simulink model "time_test"  (R2018b)
settings: Solver=VariableStepAuto  StartTime=0.0  StopTime=0  FixedStep=.2  RelTol=1e-3
values from neighbouring files (symbols this model uses):
  utc_test = 137803367    [time_test_init.m]
libraries: time_lib x1
settings Model: Creator=devantormey  LastModifiedBy=devantormey

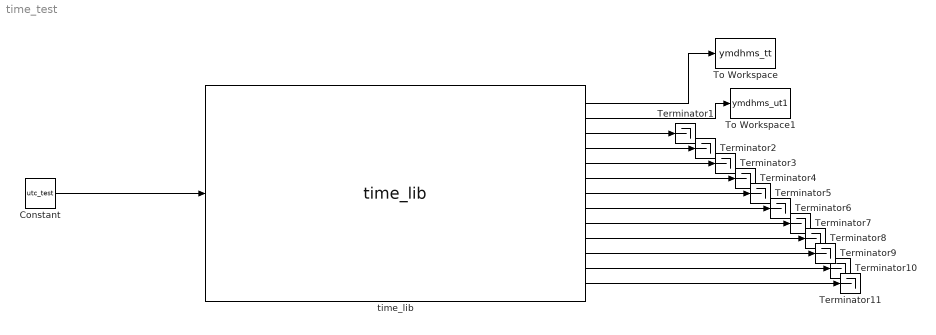
== system time_test ==
  Constant : Constant  Value=utc_test
  Terminator{1..11} (11 alike) : Terminator
  To Workspace : ToWorkspace  VariableName=ymdhms_tt  SaveFormat=Timeseries  SampleTime=-1
  To Workspace1 : ToWorkspace  VariableName=ymdhms_ut1  SaveFormat=Timeseries  SampleTime=-1
  "time_lib " : time_lib/time_lib    SystemSampleTime=-1
  wires:
  Constant/1 -> "time_lib "/1
  "time_lib "/1 -> To Workspace/1
  "time_lib "/2 -> To Workspace1/1
  "time_lib "/3 -> Terminator1/1
  "time_lib "/4 -> Terminator2/1
  "time_lib "/5 -> Terminator3/1
  "time_lib "/6 -> Terminator4/1
  "time_lib "/7 -> Terminator5/1
  "time_lib "/8 -> Terminator6/1
  "time_lib "/9 -> Terminator7/1
  "time_lib "/10 -> Terminator8/1
  "time_lib "/11 -> Terminator9/1
  "time_lib "/12 -> Terminator10/1
  "time_lib "/13 -> Terminator11/1
